simulink model "FuzzyPID"  (R2017a)
settings: Solver=VariableStepAuto  StartTime=0.0  StopTime=100.0  RelTol=1e-3
libraries: fuzblock x3, simulink x1
settings Model: Creator=Aaa  LastModifiedBy=Aaa

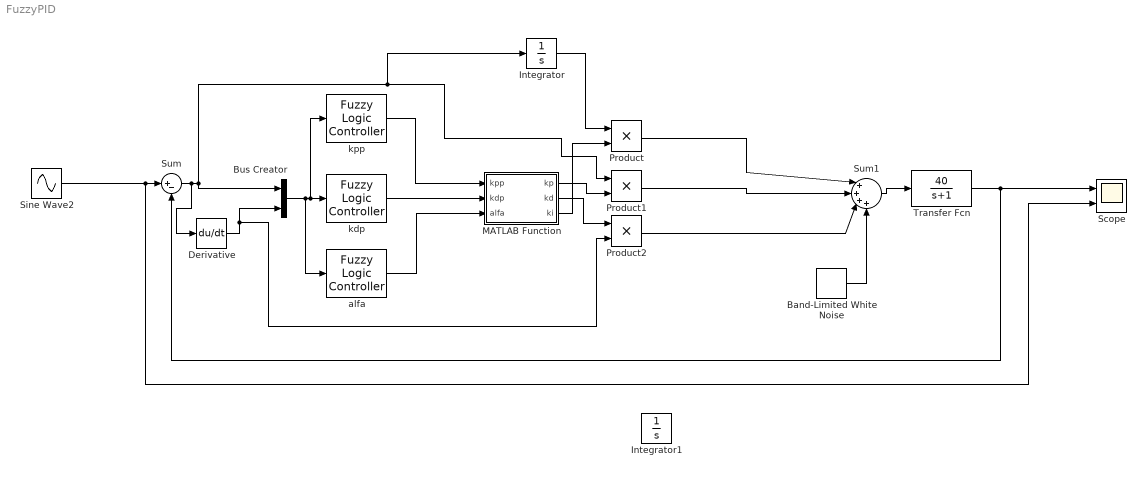
== system FuzzyPID ==
  Band-Limited White Noise : simulink/Sources/Band-Limited White Noise  Cov=[0.1]  Ts=0.1  seed=[23341]
  Bus Creator : BusCreator  Inputs=2
  Derivative : Derivative
  Integrator : Integrator
  Integrator1 : Integrator
  MATLAB Function : MATLAB Function  TreatAsAtomicUnit=on
  Product : Product
  Product1 : Product
  Product2 : Product
  Scope : Scope  NumInputPorts=2
  Sine Wave2 : Sin  SampleTime=0
  Sum : Sum  Inputs=|+-
  Sum1 : Sum  Inputs=|++++
  Transfer Fcn : TransferFcn  Numerator=[40]  Denominator=[1 1]
  alfa : fuzblock/Fuzzy Logic  Controller  fis='alfa.fis'
  kdp : fuzblock/Fuzzy Logic  Controller  fis='kdp.fis'
  kpp : fuzblock/Fuzzy Logic  Controller  fis='kpp.fis'
  wires:
  alfa/1 -> MATLAB Function/3(alfa)
  MATLAB Function/2(kd) -> Product2/1
  kdp/1 -> MATLAB Function/2(kdp)
  MATLAB Function/3(ki) -> Product/2
  Transfer Fcn/1 -> Sum/2, Scope/1
  Bus Creator/1 -> kdp/1, kpp/1, alfa/1
  Derivative/1 -> Product2/2, Bus Creator/2
  MATLAB Function/1(kp) -> Product1/2
  Sum/1 -> Derivative/1, Bus Creator/1, Integrator/1, Product1/1
  Sum1/1 -> Transfer Fcn/1
  kpp/1 -> MATLAB Function/1(kpp)
  Sine Wave2/1 -> Scope/2, Sum/1
  Product1/1 -> Sum1/2
  Product/1 -> Sum1/1
  Product2/1 -> Sum1/3
  Integrator/1 -> Product/1
  Band-Limited White Noise/1 -> Sum1/4

== matlab function FuzzyPID/MATLAB Function ==
  data: kpp input; kp output; kdp input; alfa input; kd output; ki output
function [kp,kd,ki] = fcn(kpp ,kdp,alfa)

kp=1;
kd=0;
ki=2;
% kpmin=0;
% kpmax=5;
% kdmin=0.01;
% kdmax=0.05;
% kp=kpp*(kpmax-kpmin)+kpmin;
% kd=kdp*(kdmax-kdmin)+kdmin;
% ki=(kp^2)/(alfa*kd);

% kp=1;
% kd=0;
% ki=2;
% kp = 10 *kpp;
% kd =10 *kdp +5;
% ki = (kp^2)/(alfa*kd);
